simulink model "gm_mandelbrot_fpga"  (R2019b)
settings: Solver=FixedStepDiscrete  StartTime=0.0  StopTime=33.5e-3  FixedStep=0.5*Ts  RelTol=1e-3  EnableMultiTasking=on
undefined symbols (not defined in the file or in its folder): BUTTON_CLOCK_DIV, BUTTON_DEBOUNCE, BUTTON_POLLING, LUT_BLUE, LUT_GREEN, LUT_RED, MAX_ITERATIONS, PIXEL_TIME, TRASLATION_FACTOR, Ts, VGA_HORIZONTAL_BACK_PORCH, VGA_HORIZONTAL_FRONT_PORCH, VGA_HORIZONTAL_RESOLUTION, VGA_HORIZONTAL_SYNC, VGA_VERTICAL_BACK_PORCH, VGA_VERTICAL_FRONT_PORCH, VGA_VERTICAL_RESOLUTION, VGA_VERTICAL_SYNC, ZOOM_FACTOR
libraries: simulink x132, hdlsllib x20, visionsinks x1
(part 9 of 9)

== system gm_mandelbrot_fpga/mandelbrot_top/mandelbrot_core/mandelbroot_pipeline/mandelbroot_array_instance95 ==
  stop_in : Inport  OutDataTypeStr=boolean  PortDimensions=1  SampleTime=1.35e-08
  z_in : Inport  Port=2  OutDataTypeStr=fixdt(1, 18, 15)  PortDimensions=1  SampleTime=1.35e-08
      settings: SignalType=complex
  c_in : Inport  Port=3  OutDataTypeStr=fixdt(1, 18, 15)  PortDimensions=1  SampleTime=1.35e-08
      settings: SignalType=complex
  i_in : Inport  Port=4  OutDataTypeStr=fixdt(0, 7, 0)  PortDimensions=1  SampleTime=1.35e-08
  Add : Sum
  Add1 : Sum  Inputs=+-  OutDataTypeStr=Inherit: Same as first input
  Compare To Constant : simulink/Logic and Bit Operations/Compare To Constant  relop=>=  const=4  OutDataTypeStr=boolean
  Complex to Real-Imag : ComplexToRealImag
  Constant : Constant  OutDataTypeStr=uint8  SampleTime=-1
  Data Type Conversion2 : DataTypeConversion
  Gain : Gain  Gain=2  OutDataTypeStr=Inherit: Same as input  ParamDataTypeStr=Inherit: Same as input
  Logical Operator : Logic  Operator=OR  IconShape=distinctive  AllPortsSameDT=off  OutDataTypeStr=boolean
  Product1 : Product
  Product2 : Product
  Product3 : Product
  Real-Imag to Complex : RealImagToComplex
  Sum : Sum  Inputs=|++  OutDataTypeStr=Inherit: Same as first input
  Sum1 : Sum  Inputs=|++
  Switch : Switch  Criteria=u2 ~= 0
  stop_out : Outport  VectorParamsAs1DForOutWhenUnconnected=off
  z_out : Outport  Port=2  VectorParamsAs1DForOutWhenUnconnected=off
  c_out : Outport  Port=3  VectorParamsAs1DForOutWhenUnconnected=off
  i_out : Outport  Port=4  VectorParamsAs1DForOutWhenUnconnected=off
  wires:
  i_in/1 -> Switch/1, Sum1/1
  c_in/1 -> c_out/1, Sum/2
  z_in/1 -> Complex to Real-Imag/1
  stop_in/1 -> Logical Operator/1
  Add/1 -> Compare To Constant/1
  Add1/1 -> Real-Imag to Complex/1
  Compare To Constant/1 -> Logical Operator/2
  Complex to Real-Imag/2 -> Product3/2, Product2/1, Product2/2
  Complex to Real-Imag/1 -> Product3/1, Product1/1, Product1/2
  Constant/1 -> Sum1/2
  Data Type Conversion2/1 -> z_out/1
  Gain/1 -> Real-Imag to Complex/2
  Logical Operator/1 -> stop_out/1, Switch/2
  Product1/1 -> Add1/1, Add/1
  Product2/1 -> Add1/2, Add/2
  Product3/1 -> Gain/1
  Real-Imag to Complex/1 -> Sum/1
  Sum/1 -> Data Type Conversion2/1
  Sum1/1 -> Switch/3
  Switch/1 -> i_out/1

== system gm_mandelbrot_fpga/mandelbrot_top/mandelbrot_core/mandelbroot_pipeline/mandelbroot_array_instance96 ==
  stop_in : Inport  OutDataTypeStr=boolean  PortDimensions=1  SampleTime=1.35e-08
  z_in : Inport  Port=2  OutDataTypeStr=fixdt(1, 18, 15)  PortDimensions=1  SampleTime=1.35e-08
      settings: SignalType=complex
  c_in : Inport  Port=3  OutDataTypeStr=fixdt(1, 18, 15)  PortDimensions=1  SampleTime=1.35e-08
      settings: SignalType=complex
  i_in : Inport  Port=4  OutDataTypeStr=fixdt(0, 7, 0)  PortDimensions=1  SampleTime=1.35e-08
  Add : Sum
  Add1 : Sum  Inputs=+-  OutDataTypeStr=Inherit: Same as first input
  Compare To Constant : simulink/Logic and Bit Operations/Compare To Constant  relop=>=  const=4  OutDataTypeStr=boolean
  Complex to Real-Imag : ComplexToRealImag
  Constant : Constant  OutDataTypeStr=uint8  SampleTime=-1
  Data Type Conversion2 : DataTypeConversion
  Gain : Gain  Gain=2  OutDataTypeStr=Inherit: Same as input  ParamDataTypeStr=Inherit: Same as input
  Logical Operator : Logic  Operator=OR  IconShape=distinctive  AllPortsSameDT=off  OutDataTypeStr=boolean
  Product1 : Product
  Product2 : Product
  Product3 : Product
  Real-Imag to Complex : RealImagToComplex
  Sum : Sum  Inputs=|++  OutDataTypeStr=Inherit: Same as first input
  Sum1 : Sum  Inputs=|++
  Switch : Switch  Criteria=u2 ~= 0
  stop_out : Outport  VectorParamsAs1DForOutWhenUnconnected=off
  z_out : Outport  Port=2  VectorParamsAs1DForOutWhenUnconnected=off
  c_out : Outport  Port=3  VectorParamsAs1DForOutWhenUnconnected=off
  i_out : Outport  Port=4  VectorParamsAs1DForOutWhenUnconnected=off
  wires:
  i_in/1 -> Switch/1, Sum1/1
  c_in/1 -> c_out/1, Sum/2
  z_in/1 -> Complex to Real-Imag/1
  stop_in/1 -> Logical Operator/1
  Add/1 -> Compare To Constant/1
  Add1/1 -> Real-Imag to Complex/1
  Compare To Constant/1 -> Logical Operator/2
  Complex to Real-Imag/2 -> Product3/2, Product2/1, Product2/2
  Complex to Real-Imag/1 -> Product3/1, Product1/1, Product1/2
  Constant/1 -> Sum1/2
  Data Type Conversion2/1 -> z_out/1
  Gain/1 -> Real-Imag to Complex/2
  Logical Operator/1 -> stop_out/1, Switch/2
  Product1/1 -> Add1/1, Add/1
  Product2/1 -> Add1/2, Add/2
  Product3/1 -> Gain/1
  Real-Imag to Complex/1 -> Sum/1
  Sum/1 -> Data Type Conversion2/1
  Sum1/1 -> Switch/3
  Switch/1 -> i_out/1

== system gm_mandelbrot_fpga/mandelbrot_top/mandelbrot_core/mandelbroot_pipeline/mandelbroot_array_instance97 ==
  stop_in : Inport  OutDataTypeStr=boolean  PortDimensions=1  SampleTime=1.35e-08
  z_in : Inport  Port=2  OutDataTypeStr=fixdt(1, 18, 15)  PortDimensions=1  SampleTime=1.35e-08
      settings: SignalType=complex
  c_in : Inport  Port=3  OutDataTypeStr=fixdt(1, 18, 15)  PortDimensions=1  SampleTime=1.35e-08
      settings: SignalType=complex
  i_in : Inport  Port=4  OutDataTypeStr=fixdt(0, 7, 0)  PortDimensions=1  SampleTime=1.35e-08
  Add : Sum
  Add1 : Sum  Inputs=+-  OutDataTypeStr=Inherit: Same as first input
  Compare To Constant : simulink/Logic and Bit Operations/Compare To Constant  relop=>=  const=4  OutDataTypeStr=boolean
  Complex to Real-Imag : ComplexToRealImag
  Constant : Constant  OutDataTypeStr=uint8  SampleTime=-1
  Data Type Conversion2 : DataTypeConversion
  Gain : Gain  Gain=2  OutDataTypeStr=Inherit: Same as input  ParamDataTypeStr=Inherit: Same as input
  Logical Operator : Logic  Operator=OR  IconShape=distinctive  AllPortsSameDT=off  OutDataTypeStr=boolean
  Product1 : Product
  Product2 : Product
  Product3 : Product
  Real-Imag to Complex : RealImagToComplex
  Sum : Sum  Inputs=|++  OutDataTypeStr=Inherit: Same as first input
  Sum1 : Sum  Inputs=|++
  Switch : Switch  Criteria=u2 ~= 0
  stop_out : Outport  VectorParamsAs1DForOutWhenUnconnected=off
  z_out : Outport  Port=2  VectorParamsAs1DForOutWhenUnconnected=off
  c_out : Outport  Port=3  VectorParamsAs1DForOutWhenUnconnected=off
  i_out : Outport  Port=4  VectorParamsAs1DForOutWhenUnconnected=off
  wires:
  i_in/1 -> Switch/1, Sum1/1
  c_in/1 -> c_out/1, Sum/2
  z_in/1 -> Complex to Real-Imag/1
  stop_in/1 -> Logical Operator/1
  Add/1 -> Compare To Constant/1
  Add1/1 -> Real-Imag to Complex/1
  Compare To Constant/1 -> Logical Operator/2
  Complex to Real-Imag/2 -> Product3/2, Product2/1, Product2/2
  Complex to Real-Imag/1 -> Product3/1, Product1/1, Product1/2
  Constant/1 -> Sum1/2
  Data Type Conversion2/1 -> z_out/1
  Gain/1 -> Real-Imag to Complex/2
  Logical Operator/1 -> stop_out/1, Switch/2
  Product1/1 -> Add1/1, Add/1
  Product2/1 -> Add1/2, Add/2
  Product3/1 -> Gain/1
  Real-Imag to Complex/1 -> Sum/1
  Sum/1 -> Data Type Conversion2/1
  Sum1/1 -> Switch/3
  Switch/1 -> i_out/1

== system gm_mandelbrot_fpga/mandelbrot_top/mandelbrot_core/mandelbroot_pipeline/mandelbroot_array_instance98 ==
  stop_in : Inport  OutDataTypeStr=boolean  PortDimensions=1  SampleTime=1.35e-08
  z_in : Inport  Port=2  OutDataTypeStr=fixdt(1, 18, 15)  PortDimensions=1  SampleTime=1.35e-08
      settings: SignalType=complex
  c_in : Inport  Port=3  OutDataTypeStr=fixdt(1, 18, 15)  PortDimensions=1  SampleTime=1.35e-08
      settings: SignalType=complex
  i_in : Inport  Port=4  OutDataTypeStr=fixdt(0, 7, 0)  PortDimensions=1  SampleTime=1.35e-08
  Add : Sum
  Add1 : Sum  Inputs=+-  OutDataTypeStr=Inherit: Same as first input
  Compare To Constant : simulink/Logic and Bit Operations/Compare To Constant  relop=>=  const=4  OutDataTypeStr=boolean
  Complex to Real-Imag : ComplexToRealImag
  Constant : Constant  OutDataTypeStr=uint8  SampleTime=-1
  Data Type Conversion2 : DataTypeConversion
  Gain : Gain  Gain=2  OutDataTypeStr=Inherit: Same as input  ParamDataTypeStr=Inherit: Same as input
  Logical Operator : Logic  Operator=OR  IconShape=distinctive  AllPortsSameDT=off  OutDataTypeStr=boolean
  Product1 : Product
  Product2 : Product
  Product3 : Product
  Real-Imag to Complex : RealImagToComplex
  Sum : Sum  Inputs=|++  OutDataTypeStr=Inherit: Same as first input
  Sum1 : Sum  Inputs=|++
  Switch : Switch  Criteria=u2 ~= 0
  stop_out : Outport  VectorParamsAs1DForOutWhenUnconnected=off
  z_out : Outport  Port=2  VectorParamsAs1DForOutWhenUnconnected=off
  c_out : Outport  Port=3  VectorParamsAs1DForOutWhenUnconnected=off
  i_out : Outport  Port=4  VectorParamsAs1DForOutWhenUnconnected=off
  wires:
  i_in/1 -> Switch/1, Sum1/1
  c_in/1 -> c_out/1, Sum/2
  z_in/1 -> Complex to Real-Imag/1
  stop_in/1 -> Logical Operator/1
  Add/1 -> Compare To Constant/1
  Add1/1 -> Real-Imag to Complex/1
  Compare To Constant/1 -> Logical Operator/2
  Complex to Real-Imag/2 -> Product3/2, Product2/1, Product2/2
  Complex to Real-Imag/1 -> Product3/1, Product1/1, Product1/2
  Constant/1 -> Sum1/2
  Data Type Conversion2/1 -> z_out/1
  Gain/1 -> Real-Imag to Complex/2
  Logical Operator/1 -> stop_out/1, Switch/2
  Product1/1 -> Add1/1, Add/1
  Product2/1 -> Add1/2, Add/2
  Product3/1 -> Gain/1
  Real-Imag to Complex/1 -> Sum/1
  Sum/1 -> Data Type Conversion2/1
  Sum1/1 -> Switch/3
  Switch/1 -> i_out/1

== system gm_mandelbrot_fpga/mandelbrot_top/mandelbrot_core/mandelbroot_pipeline/mandelbroot_array_instance99 ==
  stop_in : Inport  OutDataTypeStr=boolean  PortDimensions=1  SampleTime=1.35e-08
  z_in : Inport  Port=2  OutDataTypeStr=fixdt(1, 18, 15)  PortDimensions=1  SampleTime=1.35e-08
      settings: SignalType=complex
  c_in : Inport  Port=3  OutDataTypeStr=fixdt(1, 18, 15)  PortDimensions=1  SampleTime=1.35e-08
      settings: SignalType=complex
  i_in : Inport  Port=4  OutDataTypeStr=fixdt(0, 7, 0)  PortDimensions=1  SampleTime=1.35e-08
  Add : Sum
  Add1 : Sum  Inputs=+-  OutDataTypeStr=Inherit: Same as first input
  Compare To Constant : simulink/Logic and Bit Operations/Compare To Constant  relop=>=  const=4  OutDataTypeStr=boolean
  Complex to Real-Imag : ComplexToRealImag
  Constant : Constant  OutDataTypeStr=uint8  SampleTime=-1
  Data Type Conversion2 : DataTypeConversion
  Gain : Gain  Gain=2  OutDataTypeStr=Inherit: Same as input  ParamDataTypeStr=Inherit: Same as input
  Logical Operator : Logic  Operator=OR  IconShape=distinctive  AllPortsSameDT=off  OutDataTypeStr=boolean
  Product1 : Product
  Product2 : Product
  Product3 : Product
  Real-Imag to Complex : RealImagToComplex
  Sum : Sum  Inputs=|++  OutDataTypeStr=Inherit: Same as first input
  Sum1 : Sum  Inputs=|++
  Switch : Switch  Criteria=u2 ~= 0
  stop_out : Outport  VectorParamsAs1DForOutWhenUnconnected=off
  z_out : Outport  Port=2  VectorParamsAs1DForOutWhenUnconnected=off
  c_out : Outport  Port=3  VectorParamsAs1DForOutWhenUnconnected=off
  i_out : Outport  Port=4  VectorParamsAs1DForOutWhenUnconnected=off
  wires:
  i_in/1 -> Switch/1, Sum1/1
  c_in/1 -> c_out/1, Sum/2
  z_in/1 -> Complex to Real-Imag/1
  stop_in/1 -> Logical Operator/1
  Add/1 -> Compare To Constant/1
  Add1/1 -> Real-Imag to Complex/1
  Compare To Constant/1 -> Logical Operator/2
  Complex to Real-Imag/2 -> Product3/2, Product2/1, Product2/2
  Complex to Real-Imag/1 -> Product3/1, Product1/1, Product1/2
  Constant/1 -> Sum1/2
  Data Type Conversion2/1 -> z_out/1
  Gain/1 -> Real-Imag to Complex/2
  Logical Operator/1 -> stop_out/1, Switch/2
  Product1/1 -> Add1/1, Add/1
  Product2/1 -> Add1/2, Add/2
  Product3/1 -> Gain/1
  Real-Imag to Complex/1 -> Sum/1
  Sum/1 -> Data Type Conversion2/1
  Sum1/1 -> Switch/3
  Switch/1 -> i_out/1

== system gm_mandelbrot_fpga/mandelbrot_top/mandelbrot_core/vga_driver/horizontal_ranges ==
  "count " : Inport  OutDataTypeStr=uint16  SampleTime=1.35e-08
  resolution : Inport  Port=2  OutDataTypeStr=uint16  SampleTime=1.35e-08
  front_porch : Inport  Port=3  OutDataTypeStr=uint16  SampleTime=1.35e-08
  "sync " : Inport  Port=4  OutDataTypeStr=uint16  SampleTime=1.35e-08
  back_porch : Inport  Port=5  OutDataTypeStr=uint16  SampleTime=1.35e-08
  Add : Sum
  Add1 : Sum
  Add2 : Subsystem
  Constant : Constant  OutDataTypeStr=Inherit: Inherit via back propagation  SampleTime=-1
  Logical Operator : Logic  IconShape=distinctive  AllPortsSameDT=off  OutDataTypeStr=boolean
  Relational Operator : RelationalOperator  Operator=<  OutDataTypeStr=boolean  RndMeth=Simplest
  Relational Operator1 : RelationalOperator  OutDataTypeStr=boolean  RndMeth=Simplest
  Relational Operator2 : RelationalOperator  Operator=<  OutDataTypeStr=boolean  RndMeth=Simplest
  Relational Operator3 : RelationalOperator  Operator===  OutDataTypeStr=boolean  RndMeth=Simplest
  "index " : Outport
  "sync_pulse " : Outport  Port=2
  "eoc " : Outport  Port=3
  video_enable : Outport  Port=4
  wires:
  "count "/1 -> Relational Operator3/1, Relational Operator2/1, Relational Operator1/1, Relational Operator/1, "index "/1
  resolution/1 -> Relational Operator/2, Add/1
  front_porch/1 -> Add/2
  "sync "/1 -> Add1/2
  back_porch/1 -> Add2/2(In2)
  Add/1 -> Relational Operator1/2, Add1/1
  Add1/1 -> Relational Operator2/2, Add2/1(In1)
  Add2/1(Out1) -> Relational Operator3/2
  Constant/1 -> Add2/3(In3)
  Logical Operator/1 -> "sync_pulse "/1
  Relational Operator/1 -> video_enable/1
  Relational Operator1/1 -> Logical Operator/1
  Relational Operator2/1 -> Logical Operator/2
  Relational Operator3/1 -> "eoc "/1

== system gm_mandelbrot_fpga/mandelbrot_top/mandelbrot_core/vga_driver/vertical_ranges  ==
  "count " : Inport  OutDataTypeStr=uint16  SampleTime=1.35e-08
  resolution : Inport  Port=2  OutDataTypeStr=uint16  SampleTime=1.35e-08
  front_porch : Inport  Port=3  OutDataTypeStr=uint16  SampleTime=1.35e-08
  "sync " : Inport  Port=4  OutDataTypeStr=uint16  SampleTime=1.35e-08
  back_porch : Inport  Port=5  OutDataTypeStr=uint16  SampleTime=1.35e-08
  Add : Sum
  Add1 : Sum
  Logical Operator : Logic  IconShape=distinctive  AllPortsSameDT=off  OutDataTypeStr=boolean
  Relational Operator : RelationalOperator  Operator=<  OutDataTypeStr=boolean  RndMeth=Simplest
  Relational Operator1 : RelationalOperator  OutDataTypeStr=boolean  RndMeth=Simplest
  Relational Operator2 : RelationalOperator  Operator=<  OutDataTypeStr=boolean  RndMeth=Simplest
  "index " : Outport
  "sync_pulse " : Outport  Port=2
  video_enable : Outport  Port=3
  wires:
  "count "/1 -> Relational Operator2/1, Relational Operator1/1, Relational Operator/1, "index "/1
  resolution/1 -> Relational Operator/2, Add/1
  front_porch/1 -> Add/2
  "sync "/1 -> Add1/2
  Add/1 -> Relational Operator1/2, Add1/1
  Add1/1 -> Relational Operator2/2
  Logical Operator/1 -> "sync_pulse "/1
  Relational Operator/1 -> video_enable/1
  Relational Operator1/1 -> Logical Operator/1
  Relational Operator2/1 -> Logical Operator/2

== system gm_mandelbrot_fpga/mandelbrot_top/mandelbrot_core/vga_driver/horizontal_ranges/Add2 ==
  In1 : Inport  OutDataTypeStr=fixdt(0,18,0)
  In2 : Inport  Port=2  OutDataTypeStr=fixdt(0,16,0)
  In3 : Inport  Port=3  OutDataTypeStr=fixdt(0,18,0)
  Sum2 : Sum  AccumDataTypeStr=fixdt(1,20,0)  OutDataTypeStr=fixdt(1,20,0)
  Sum3 : Sum  Inputs=+-  AccumDataTypeStr=fixdt(1,20,0)  OutDataTypeStr=fixdt(1,20,0)
  Out1 : Outport
  wires:
  In1/1 -> Sum2/1
  In2/1 -> Sum2/2
  Sum2/1 -> Sum3/1
  In3/1 -> Sum3/2
  Sum3/1 -> Out1/1

== matlab function gm_mandelbrot_fpga/vga_screen/handle_video_matrix ==
  data: video_matrix_in input; video_matrix_out output; x input; y input; red input; green input; blue input; max_x input; max_y input
function video_matrix_out = handle_video_matrix(video_matrix_in, x, y, red, green, blue, max_x, max_y)
%#codegen

temp = video_matrix_in;
if x <= max_x && y <= max_y 
    temp(y, x, :) = [double(red)/255.0 double(green)/255.0 double(blue)/255.0];
end
video_matrix_out = temp;
